simulink model "c00006M_harness"  (R2018a)
settings: Solver=FixedStepAuto  StartTime=0.0  StopTime=300  FixedStep=0.1  RelTol=1e-3
undefined symbols (not defined in the file): A1, hmax, PriorityTank, R1, R2, sigbuilder_block, TempThreshold
(part 6 of 66)

== system c00006M_harness/M105 ==
  note: VALUES
      | ---------------------------------
      | ControlType = 1 | 2 | 3
      | FillTank = 0 | 1
      | EmptyTank = 0 | 1
      | ManualReference between 0 and 1
      | Tempreature between 0 and 100
      | EmergencyButton = 0 | 1
      | LiquidLevel between 0 and 1 (hmax)
  note: Inputs For Tank2
  note: NAMES
      | --------------------------------------------
      | CT1 = ControlType Tank 1
      | F1 = Fill Tank 1
      | E1 = Empty Tank 1
      | MR1 = Manual Reference Tank1
      | T1 = Temperature Tank 1
      | EB1 = Emergency Button Tank 1
      | LL1 = Liquid Level 1
  note: Inputs For Tank3
  note: Inputs For Tank1
  CT2 : Inport
  F2 : Inport  Port=2
  E2 : Inport  Port=3
  MR2 : Inport  Port=4
  T2 : Inport  Port=5
  EB2 : Inport  Port=6
  CT3 : Inport  Port=7
  F3 : Inport  Port=8
  E3 : Inport  Port=9
  MR3 : Inport  Port=10
  T3 : Inport  Port=11
  EB3 : Inport  Port=12
  Tank2 : Subsystem
  Tank3 : Subsystem
  LL2 : Outport
  LL3 : Outport  Port=2
  wires:
  Tank2/1(LL2) -> LL2/1, Tank3/7(LL2)
  Tank3/1(LL3) -> LL3/1, Tank2/7(LL3)
  EB2/1 -> Tank2/6(EB2)
  MR3/1 -> Tank3/4(MR3)
  CT2/1 -> Tank2/1(CT2)
  F2/1 -> Tank2/2(F2)
  E3/1 -> Tank3/3(E3)
  E2/1 -> Tank2/3(E2)
  T2/1 -> Tank2/5(T2)
  CT3/1 -> Tank3/1(CT3)
  F3/1 -> Tank3/2(F3)
  EB3/1 -> Tank3/6(EB3)
  T3/1 -> Tank3/5(T3)
  MR2/1 -> Tank2/4(MR2)

== system c00006M_harness/M106 ==
  note: VALUES
      | ---------------------------------
      | ControlType = 1 | 2 | 3
      | FillTank = 0 | 1
      | EmptyTank = 0 | 1
      | ManualReference between 0 and 1
      | Tempreature between 0 and 100
      | EmergencyButton = 0 | 1
      | LiquidLevel between 0 and 1 (hmax)
  note: Inputs For Tank2
  note: NAMES
      | --------------------------------------------
      | CT1 = ControlType Tank 1
      | F1 = Fill Tank 1
      | E1 = Empty Tank 1
      | MR1 = Manual Reference Tank1
      | T1 = Temperature Tank 1
      | EB1 = Emergency Button Tank 1
      | LL1 = Liquid Level 1
  note: Inputs For Tank3
  note: Inputs For Tank1
  CT2 : Inport
  F2 : Inport  Port=2
  E2 : Inport  Port=3
  MR2 : Inport  Port=4
  T2 : Inport  Port=5
  EB2 : Inport  Port=6
  CT3 : Inport  Port=7
  F3 : Inport  Port=8
  E3 : Inport  Port=9
  MR3 : Inport  Port=10
  T3 : Inport  Port=11
  EB3 : Inport  Port=12
  Tank2 : Subsystem
  Tank3 : Subsystem
  LL2 : Outport
  LL3 : Outport  Port=2
  wires:
  Tank2/1(LL2) -> LL2/1, Tank3/7(LL2)
  Tank3/1(LL3) -> LL3/1, Tank2/7(LL3)
  EB2/1 -> Tank2/6(EB2)
  MR3/1 -> Tank3/4(MR3)
  CT2/1 -> Tank2/1(CT2)
  F2/1 -> Tank2/2(F2)
  E3/1 -> Tank3/3(E3)
  E2/1 -> Tank2/3(E2)
  T2/1 -> Tank2/5(T2)
  CT3/1 -> Tank3/1(CT3)
  F3/1 -> Tank3/2(F3)
  EB3/1 -> Tank3/6(EB3)
  T3/1 -> Tank3/5(T3)
  MR2/1 -> Tank2/4(MR2)

== system c00006M_harness/M107 ==
  note: VALUES
      | ---------------------------------
      | ControlType = 1 | 2 | 3
      | FillTank = 0 | 1
      | EmptyTank = 0 | 1
      | ManualReference between 0 and 1
      | Tempreature between 0 and 100
      | EmergencyButton = 0 | 1
      | LiquidLevel between 0 and 1 (hmax)
  note: Inputs For Tank2
  note: NAMES
      | --------------------------------------------
      | CT1 = ControlType Tank 1
      | F1 = Fill Tank 1
      | E1 = Empty Tank 1
      | MR1 = Manual Reference Tank1
      | T1 = Temperature Tank 1
      | EB1 = Emergency Button Tank 1
      | LL1 = Liquid Level 1
  note: Inputs For Tank3
  note: Inputs For Tank1
  CT2 : Inport
  F2 : Inport  Port=2
  E2 : Inport  Port=3
  MR2 : Inport  Port=4
  T2 : Inport  Port=5
  EB2 : Inport  Port=6
  CT3 : Inport  Port=7
  F3 : Inport  Port=8
  E3 : Inport  Port=9
  MR3 : Inport  Port=10
  T3 : Inport  Port=11
  EB3 : Inport  Port=12
  Tank2 : Subsystem
  Tank3 : Subsystem
  LL2 : Outport
  LL3 : Outport  Port=2
  wires:
  Tank2/1(LL2) -> LL2/1, Tank3/7(LL2)
  Tank3/1(LL3) -> LL3/1, Tank2/7(LL3)
  EB2/1 -> Tank2/6(EB2)
  MR3/1 -> Tank3/4(MR3)
  CT2/1 -> Tank2/1(CT2)
  F2/1 -> Tank2/2(F2)
  E3/1 -> Tank3/3(E3)
  E2/1 -> Tank2/3(E2)
  T2/1 -> Tank2/5(T2)
  CT3/1 -> Tank3/1(CT3)
  F3/1 -> Tank3/2(F3)
  EB3/1 -> Tank3/6(EB3)
  T3/1 -> Tank3/5(T3)
  MR2/1 -> Tank2/4(MR2)

== system c00006M_harness/M108 ==
  note: VALUES
      | ---------------------------------
      | ControlType = 1 | 2 | 3
      | FillTank = 0 | 1
      | EmptyTank = 0 | 1
      | ManualReference between 0 and 1
      | Tempreature between 0 and 100
      | EmergencyButton = 0 | 1
      | LiquidLevel between 0 and 1 (hmax)
  note: Inputs For Tank2
  note: NAMES
      | --------------------------------------------
      | CT1 = ControlType Tank 1
      | F1 = Fill Tank 1
      | E1 = Empty Tank 1
      | MR1 = Manual Reference Tank1
      | T1 = Temperature Tank 1
      | EB1 = Emergency Button Tank 1
      | LL1 = Liquid Level 1
  note: Inputs For Tank3
  note: Inputs For Tank1
  CT2 : Inport
  F2 : Inport  Port=2
  E2 : Inport  Port=3
  MR2 : Inport  Port=4
  T2 : Inport  Port=5
  EB2 : Inport  Port=6
  CT3 : Inport  Port=7
  F3 : Inport  Port=8
  E3 : Inport  Port=9
  MR3 : Inport  Port=10
  T3 : Inport  Port=11
  EB3 : Inport  Port=12
  Tank2 : Subsystem
  Tank3 : Subsystem
  LL2 : Outport
  LL3 : Outport  Port=2
  wires:
  Tank2/1(LL2) -> LL2/1, Tank3/7(LL2)
  Tank3/1(LL3) -> LL3/1, Tank2/7(LL3)
  EB2/1 -> Tank2/6(EB2)
  MR3/1 -> Tank3/4(MR3)
  CT2/1 -> Tank2/1(CT2)
  F2/1 -> Tank2/2(F2)
  E3/1 -> Tank3/3(E3)
  E2/1 -> Tank2/3(E2)
  T2/1 -> Tank2/5(T2)
  CT3/1 -> Tank3/1(CT3)
  F3/1 -> Tank3/2(F3)
  EB3/1 -> Tank3/6(EB3)
  T3/1 -> Tank3/5(T3)
  MR2/1 -> Tank2/4(MR2)

== system c00006M_harness/M109 ==
  note: VALUES
      | ---------------------------------
      | ControlType = 1 | 2 | 3
      | FillTank = 0 | 1
      | EmptyTank = 0 | 1
      | ManualReference between 0 and 1
      | Tempreature between 0 and 100
      | EmergencyButton = 0 | 1
      | LiquidLevel between 0 and 1 (hmax)
  note: Inputs For Tank2
  note: NAMES
      | --------------------------------------------
      | CT1 = ControlType Tank 1
      | F1 = Fill Tank 1
      | E1 = Empty Tank 1
      | MR1 = Manual Reference Tank1
      | T1 = Temperature Tank 1
      | EB1 = Emergency Button Tank 1
      | LL1 = Liquid Level 1
  note: Inputs For Tank3
  note: Inputs For Tank1
  CT2 : Inport
  F2 : Inport  Port=2
  E2 : Inport  Port=3
  MR2 : Inport  Port=4
  T2 : Inport  Port=5
  EB2 : Inport  Port=6
  CT3 : Inport  Port=7
  F3 : Inport  Port=8
  E3 : Inport  Port=9
  MR3 : Inport  Port=10
  T3 : Inport  Port=11
  EB3 : Inport  Port=12
  Tank2 : Subsystem
  Tank3 : Subsystem
  LL2 : Outport
  LL3 : Outport  Port=2
  wires:
  Tank2/1(LL2) -> LL2/1, Tank3/7(LL2)
  Tank3/1(LL3) -> LL3/1, Tank2/7(LL3)
  EB2/1 -> Tank2/6(EB2)
  MR3/1 -> Tank3/4(MR3)
  CT2/1 -> Tank2/1(CT2)
  F2/1 -> Tank2/2(F2)
  E3/1 -> Tank3/3(E3)
  E2/1 -> Tank2/3(E2)
  T2/1 -> Tank2/5(T2)
  CT3/1 -> Tank3/1(CT3)
  F3/1 -> Tank3/2(F3)
  EB3/1 -> Tank3/6(EB3)
  T3/1 -> Tank3/5(T3)
  MR2/1 -> Tank2/4(MR2)

== system c00006M_harness/M110 ==
  note: VALUES
      | ---------------------------------
      | ControlType = 1 | 2 | 3
      | FillTank = 0 | 1
      | EmptyTank = 0 | 1
      | ManualReference between 0 and 1
      | Tempreature between 0 and 100
      | EmergencyButton = 0 | 1
      | LiquidLevel between 0 and 1 (hmax)
  note: Inputs For Tank2
  note: NAMES
      | --------------------------------------------
      | CT1 = ControlType Tank 1
      | F1 = Fill Tank 1
      | E1 = Empty Tank 1
      | MR1 = Manual Reference Tank1
      | T1 = Temperature Tank 1
      | EB1 = Emergency Button Tank 1
      | LL1 = Liquid Level 1
  note: Inputs For Tank3
  note: Inputs For Tank1
  CT2 : Inport
  F2 : Inport  Port=2
  E2 : Inport  Port=3
  MR2 : Inport  Port=4
  T2 : Inport  Port=5
  EB2 : Inport  Port=6
  CT3 : Inport  Port=7
  F3 : Inport  Port=8
  E3 : Inport  Port=9
  MR3 : Inport  Port=10
  T3 : Inport  Port=11
  EB3 : Inport  Port=12
  Tank2 : Subsystem
  Tank3 : Subsystem
  LL2 : Outport
  LL3 : Outport  Port=2
  wires:
  Tank2/1(LL2) -> LL2/1, Tank3/7(LL2)
  Tank3/1(LL3) -> LL3/1, Tank2/7(LL3)
  EB2/1 -> Tank2/6(EB2)
  MR3/1 -> Tank3/4(MR3)
  CT2/1 -> Tank2/1(CT2)
  F2/1 -> Tank2/2(F2)
  E3/1 -> Tank3/3(E3)
  E2/1 -> Tank2/3(E2)
  T2/1 -> Tank2/5(T2)
  CT3/1 -> Tank3/1(CT3)
  F3/1 -> Tank3/2(F3)
  EB3/1 -> Tank3/6(EB3)
  T3/1 -> Tank3/5(T3)
  MR2/1 -> Tank2/4(MR2)

== system c00006M_harness/M111 ==
  note: VALUES
      | ---------------------------------
      | ControlType = 1 | 2 | 3
      | FillTank = 0 | 1
      | EmptyTank = 0 | 1
      | ManualReference between 0 and 1
      | Tempreature between 0 and 100
      | EmergencyButton = 0 | 1
      | LiquidLevel between 0 and 1 (hmax)
  note: Inputs For Tank2
  note: NAMES
      | --------------------------------------------
      | CT1 = ControlType Tank 1
      | F1 = Fill Tank 1
      | E1 = Empty Tank 1
      | MR1 = Manual Reference Tank1
      | T1 = Temperature Tank 1
      | EB1 = Emergency Button Tank 1
      | LL1 = Liquid Level 1
  note: Inputs For Tank3
  note: Inputs For Tank1
  CT2 : Inport
  F2 : Inport  Port=2
  E2 : Inport  Port=3
  MR2 : Inport  Port=4
  T2 : Inport  Port=5
  EB2 : Inport  Port=6
  CT3 : Inport  Port=7
  F3 : Inport  Port=8
  E3 : Inport  Port=9
  MR3 : Inport  Port=10
  T3 : Inport  Port=11
  EB3 : Inport  Port=12
  Tank2 : Subsystem
  Tank3 : Subsystem
  LL2 : Outport
  LL3 : Outport  Port=2
  wires:
  Tank2/1(LL2) -> LL2/1, Tank3/7(LL2)
  Tank3/1(LL3) -> LL3/1, Tank2/7(LL3)
  EB2/1 -> Tank2/6(EB2)
  MR3/1 -> Tank3/4(MR3)
  CT2/1 -> Tank2/1(CT2)
  F2/1 -> Tank2/2(F2)
  E3/1 -> Tank3/3(E3)
  E2/1 -> Tank2/3(E2)
  T2/1 -> Tank2/5(T2)
  CT3/1 -> Tank3/1(CT3)
  F3/1 -> Tank3/2(F3)
  EB3/1 -> Tank3/6(EB3)
  T3/1 -> Tank3/5(T3)
  MR2/1 -> Tank2/4(MR2)

== system c00006M_harness/M112 ==
  note: VALUES
      | ---------------------------------
      | ControlType = 1 | 2 | 3
      | FillTank = 0 | 1
      | EmptyTank = 0 | 1
      | ManualReference between 0 and 1
      | Tempreature between 0 and 100
      | EmergencyButton = 0 | 1
      | LiquidLevel between 0 and 1 (hmax)
  note: Inputs For Tank2
  note: NAMES
      | --------------------------------------------
      | CT1 = ControlType Tank 1
      | F1 = Fill Tank 1
      | E1 = Empty Tank 1
      | MR1 = Manual Reference Tank1
      | T1 = Temperature Tank 1
      | EB1 = Emergency Button Tank 1
      | LL1 = Liquid Level 1
  note: Inputs For Tank3
  note: Inputs For Tank1
  CT2 : Inport
  F2 : Inport  Port=2
  E2 : Inport  Port=3
  MR2 : Inport  Port=4
  T2 : Inport  Port=5
  EB2 : Inport  Port=6
  CT3 : Inport  Port=7
  F3 : Inport  Port=8
  E3 : Inport  Port=9
  MR3 : Inport  Port=10
  T3 : Inport  Port=11
  EB3 : Inport  Port=12
  Tank2 : Subsystem
  Tank3 : Subsystem
  LL2 : Outport
  LL3 : Outport  Port=2
  wires:
  Tank2/1(LL2) -> LL2/1, Tank3/7(LL2)
  Tank3/1(LL3) -> LL3/1, Tank2/7(LL3)
  EB2/1 -> Tank2/6(EB2)
  MR3/1 -> Tank3/4(MR3)
  CT2/1 -> Tank2/1(CT2)
  F2/1 -> Tank2/2(F2)
  E3/1 -> Tank3/3(E3)
  E2/1 -> Tank2/3(E2)
  T2/1 -> Tank2/5(T2)
  CT3/1 -> Tank3/1(CT3)
  F3/1 -> Tank3/2(F3)
  EB3/1 -> Tank3/6(EB3)
  T3/1 -> Tank3/5(T3)
  MR2/1 -> Tank2/4(MR2)

== system c00006M_harness/M113 ==
  note: VALUES
      | ---------------------------------
      | ControlType = 1 | 2 | 3
      | FillTank = 0 | 1
      | EmptyTank = 0 | 1
      | ManualReference between 0 and 1
      | Tempreature between 0 and 100
      | EmergencyButton = 0 | 1
      | LiquidLevel between 0 and 1 (hmax)
  note: Inputs For Tank2
  note: NAMES
      | --------------------------------------------
      | CT1 = ControlType Tank 1
      | F1 = Fill Tank 1
      | E1 = Empty Tank 1
      | MR1 = Manual Reference Tank1
      | T1 = Temperature Tank 1
      | EB1 = Emergency Button Tank 1
      | LL1 = Liquid Level 1
  note: Inputs For Tank3
  note: Inputs For Tank1
  CT2 : Inport
  F2 : Inport  Port=2
  E2 : Inport  Port=3
  MR2 : Inport  Port=4
  T2 : Inport  Port=5
  EB2 : Inport  Port=6
  CT3 : Inport  Port=7
  F3 : Inport  Port=8
  E3 : Inport  Port=9
  MR3 : Inport  Port=10
  T3 : Inport  Port=11
  EB3 : Inport  Port=12
  Tank2 : Subsystem
  Tank3 : Subsystem
  LL2 : Outport
  LL3 : Outport  Port=2
  wires:
  Tank2/1(LL2) -> LL2/1, Tank3/7(LL2)
  Tank3/1(LL3) -> LL3/1, Tank2/7(LL3)
  EB2/1 -> Tank2/6(EB2)
  MR3/1 -> Tank3/4(MR3)
  CT2/1 -> Tank2/1(CT2)
  F2/1 -> Tank2/2(F2)
  E3/1 -> Tank3/3(E3)
  E2/1 -> Tank2/3(E2)
  T2/1 -> Tank2/5(T2)
  CT3/1 -> Tank3/1(CT3)
  F3/1 -> Tank3/2(F3)
  EB3/1 -> Tank3/6(EB3)
  T3/1 -> Tank3/5(T3)
  MR2/1 -> Tank2/4(MR2)

== system c00006M_harness/M114 ==
  note: VALUES
      | ---------------------------------
      | ControlType = 1 | 2 | 3
      | FillTank = 0 | 1
      | EmptyTank = 0 | 1
      | ManualReference between 0 and 1
      | Tempreature between 0 and 100
      | EmergencyButton = 0 | 1
      | LiquidLevel between 0 and 1 (hmax)
  note: Inputs For Tank2
  note: NAMES
      | --------------------------------------------
      | CT1 = ControlType Tank 1
      | F1 = Fill Tank 1
      | E1 = Empty Tank 1
      | MR1 = Manual Reference Tank1
      | T1 = Temperature Tank 1
      | EB1 = Emergency Button Tank 1
      | LL1 = Liquid Level 1
  note: Inputs For Tank3
  note: Inputs For Tank1
  CT2 : Inport
  F2 : Inport  Port=2
  E2 : Inport  Port=3
  MR2 : Inport  Port=4
  T2 : Inport  Port=5
  EB2 : Inport  Port=6
  CT3 : Inport  Port=7
  F3 : Inport  Port=8
  E3 : Inport  Port=9
  MR3 : Inport  Port=10
  T3 : Inport  Port=11
  EB3 : Inport  Port=12
  Tank2 : Subsystem
  Tank3 : Subsystem
  LL2 : Outport
  LL3 : Outport  Port=2
  wires:
  Tank2/1(LL2) -> LL2/1, Tank3/7(LL2)
  Tank3/1(LL3) -> LL3/1, Tank2/7(LL3)
  EB2/1 -> Tank2/6(EB2)
  MR3/1 -> Tank3/4(MR3)
  CT2/1 -> Tank2/1(CT2)
  F2/1 -> Tank2/2(F2)
  E3/1 -> Tank3/3(E3)
  E2/1 -> Tank2/3(E2)
  T2/1 -> Tank2/5(T2)
  CT3/1 -> Tank3/1(CT3)
  F3/1 -> Tank3/2(F3)
  EB3/1 -> Tank3/6(EB3)
  T3/1 -> Tank3/5(T3)
  MR2/1 -> Tank2/4(MR2)

== system c00006M_harness/M115 ==
  note: VALUES
      | ---------------------------------
      | ControlType = 1 | 2 | 3
      | FillTank = 0 | 1
      | EmptyTank = 0 | 1
      | ManualReference between 0 and 1
      | Tempreature between 0 and 100
      | EmergencyButton = 0 | 1
      | LiquidLevel between 0 and 1 (hmax)
  note: Inputs For Tank2
  note: NAMES
      | --------------------------------------------
      | CT1 = ControlType Tank 1
      | F1 = Fill Tank 1
      | E1 = Empty Tank 1
      | MR1 = Manual Reference Tank1
      | T1 = Temperature Tank 1
      | EB1 = Emergency Button Tank 1
      | LL1 = Liquid Level 1
  note: Inputs For Tank3
  note: Inputs For Tank1
  CT2 : Inport
  F2 : Inport  Port=2
  E2 : Inport  Port=3
  MR2 : Inport  Port=4
  T2 : Inport  Port=5
  EB2 : Inport  Port=6
  CT3 : Inport  Port=7
  F3 : Inport  Port=8
  E3 : Inport  Port=9
  MR3 : Inport  Port=10
  T3 : Inport  Port=11
  EB3 : Inport  Port=12
  Tank2 : Subsystem
  Tank3 : Subsystem
  LL2 : Outport
  LL3 : Outport  Port=2
  wires:
  Tank2/1(LL2) -> LL2/1, Tank3/7(LL2)
  Tank3/1(LL3) -> LL3/1, Tank2/7(LL3)
  EB2/1 -> Tank2/6(EB2)
  MR3/1 -> Tank3/4(MR3)
  CT2/1 -> Tank2/1(CT2)
  F2/1 -> Tank2/2(F2)
  E3/1 -> Tank3/3(E3)
  E2/1 -> Tank2/3(E2)
  T2/1 -> Tank2/5(T2)
  CT3/1 -> Tank3/1(CT3)
  F3/1 -> Tank3/2(F3)
  EB3/1 -> Tank3/6(EB3)
  T3/1 -> Tank3/5(T3)
  MR2/1 -> Tank2/4(MR2)

== system c00006M_harness/M116 ==
  note: VALUES
      | ---------------------------------
      | ControlType = 1 | 2 | 3
      | FillTank = 0 | 1
      | EmptyTank = 0 | 1
      | ManualReference between 0 and 1
      | Tempreature between 0 and 100
      | EmergencyButton = 0 | 1
      | LiquidLevel between 0 and 1 (hmax)
  note: Inputs For Tank2
  note: NAMES
      | --------------------------------------------
      | CT1 = ControlType Tank 1
      | F1 = Fill Tank 1
      | E1 = Empty Tank 1
      | MR1 = Manual Reference Tank1
      | T1 = Temperature Tank 1
      | EB1 = Emergency Button Tank 1
      | LL1 = Liquid Level 1
  note: Inputs For Tank3
  note: Inputs For Tank1
  CT2 : Inport
  F2 : Inport  Port=2
  E2 : Inport  Port=3
  MR2 : Inport  Port=4
  T2 : Inport  Port=5
  EB2 : Inport  Port=6
  CT3 : Inport  Port=7
  F3 : Inport  Port=8
  E3 : Inport  Port=9
  MR3 : Inport  Port=10
  T3 : Inport  Port=11
  EB3 : Inport  Port=12
  Tank2 : Subsystem
  Tank3 : Subsystem
  LL2 : Outport
  LL3 : Outport  Port=2
  wires:
  Tank2/1(LL2) -> LL2/1, Tank3/7(LL2)
  Tank3/1(LL3) -> LL3/1, Tank2/7(LL3)
  EB2/1 -> Tank2/6(EB2)
  MR3/1 -> Tank3/4(MR3)
  CT2/1 -> Tank2/1(CT2)
  F2/1 -> Tank2/2(F2)
  E3/1 -> Tank3/3(E3)
  E2/1 -> Tank2/3(E2)
  T2/1 -> Tank2/5(T2)
  CT3/1 -> Tank3/1(CT3)
  F3/1 -> Tank3/2(F3)
  EB3/1 -> Tank3/6(EB3)
  T3/1 -> Tank3/5(T3)
  MR2/1 -> Tank2/4(MR2)

== system c00006M_harness/M117 ==
  note: VALUES
      | ---------------------------------
      | ControlType = 1 | 2 | 3
      | FillTank = 0 | 1
      | EmptyTank = 0 | 1
      | ManualReference between 0 and 1
      | Tempreature between 0 and 100
      | EmergencyButton = 0 | 1
      | LiquidLevel between 0 and 1 (hmax)
  note: Inputs For Tank2
  note: NAMES
      | --------------------------------------------
      | CT1 = ControlType Tank 1
      | F1 = Fill Tank 1
      | E1 = Empty Tank 1
      | MR1 = Manual Reference Tank1
      | T1 = Temperature Tank 1
      | EB1 = Emergency Button Tank 1
      | LL1 = Liquid Level 1
  note: Inputs For Tank3
  note: Inputs For Tank1
  CT2 : Inport
  F2 : Inport  Port=2
  E2 : Inport  Port=3
  MR2 : Inport  Port=4
  T2 : Inport  Port=5
  EB2 : Inport  Port=6
  CT3 : Inport  Port=7
  F3 : Inport  Port=8
  E3 : Inport  Port=9
  MR3 : Inport  Port=10
  T3 : Inport  Port=11
  EB3 : Inport  Port=12
  Tank2 : Subsystem
  Tank3 : Subsystem
  LL2 : Outport
  LL3 : Outport  Port=2
  wires:
  Tank2/1(LL2) -> LL2/1, Tank3/7(LL2)
  Tank3/1(LL3) -> LL3/1, Tank2/7(LL3)
  EB2/1 -> Tank2/6(EB2)
  MR3/1 -> Tank3/4(MR3)
  CT2/1 -> Tank2/1(CT2)
  F2/1 -> Tank2/2(F2)
  E3/1 -> Tank3/3(E3)
  E2/1 -> Tank2/3(E2)
  T2/1 -> Tank2/5(T2)
  CT3/1 -> Tank3/1(CT3)
  F3/1 -> Tank3/2(F3)
  EB3/1 -> Tank3/6(EB3)
  T3/1 -> Tank3/5(T3)
  MR2/1 -> Tank2/4(MR2)

== system c00006M_harness/M118 ==
  note: VALUES
      | ---------------------------------
      | ControlType = 1 | 2 | 3
      | FillTank = 0 | 1
      | EmptyTank = 0 | 1
      | ManualReference between 0 and 1
      | Tempreature between 0 and 100
      | EmergencyButton = 0 | 1
      | LiquidLevel between 0 and 1 (hmax)
  note: Inputs For Tank2
  note: NAMES
      | --------------------------------------------
      | CT1 = ControlType Tank 1
      | F1 = Fill Tank 1
      | E1 = Empty Tank 1
      | MR1 = Manual Reference Tank1
      | T1 = Temperature Tank 1
      | EB1 = Emergency Button Tank 1
      | LL1 = Liquid Level 1
  note: Inputs For Tank3
  note: Inputs For Tank1
  CT2 : Inport
  F2 : Inport  Port=2
  E2 : Inport  Port=3
  MR2 : Inport  Port=4
  T2 : Inport  Port=5
  EB2 : Inport  Port=6
  CT3 : Inport  Port=7
  F3 : Inport  Port=8
  E3 : Inport  Port=9
  MR3 : Inport  Port=10
  T3 : Inport  Port=11
  EB3 : Inport  Port=12
  Tank2 : Subsystem
  Tank3 : Subsystem
  LL2 : Outport
  LL3 : Outport  Port=2
  wires:
  Tank2/1(LL2) -> LL2/1, Tank3/7(LL2)
  Tank3/1(LL3) -> LL3/1, Tank2/7(LL3)
  EB2/1 -> Tank2/6(EB2)
  MR3/1 -> Tank3/4(MR3)
  CT2/1 -> Tank2/1(CT2)
  F2/1 -> Tank2/2(F2)
  E3/1 -> Tank3/3(E3)
  E2/1 -> Tank2/3(E2)
  T2/1 -> Tank2/5(T2)
  CT3/1 -> Tank3/1(CT3)
  F3/1 -> Tank3/2(F3)
  EB3/1 -> Tank3/6(EB3)
  T3/1 -> Tank3/5(T3)
  MR2/1 -> Tank2/4(MR2)

== system c00006M_harness/M119 ==
  note: VALUES
      | ---------------------------------
      | ControlType = 1 | 2 | 3
      | FillTank = 0 | 1
      | EmptyTank = 0 | 1
      | ManualReference between 0 and 1
      | Tempreature between 0 and 100
      | EmergencyButton = 0 | 1
      | LiquidLevel between 0 and 1 (hmax)
  note: Inputs For Tank2
  note: NAMES
      | --------------------------------------------
      | CT1 = ControlType Tank 1
      | F1 = Fill Tank 1
      | E1 = Empty Tank 1
      | MR1 = Manual Reference Tank1
      | T1 = Temperature Tank 1
      | EB1 = Emergency Button Tank 1
      | LL1 = Liquid Level 1
  note: Inputs For Tank3
  note: Inputs For Tank1
  CT2 : Inport
  F2 : Inport  Port=2
  E2 : Inport  Port=3
  MR2 : Inport  Port=4
  T2 : Inport  Port=5
  EB2 : Inport  Port=6
  CT3 : Inport  Port=7
  F3 : Inport  Port=8
  E3 : Inport  Port=9
  MR3 : Inport  Port=10
  T3 : Inport  Port=11
  EB3 : Inport  Port=12
  Tank2 : Subsystem
  Tank3 : Subsystem
  LL2 : Outport
  LL3 : Outport  Port=2
  wires:
  Tank2/1(LL2) -> LL2/1, Tank3/7(LL2)
  Tank3/1(LL3) -> LL3/1, Tank2/7(LL3)
  EB2/1 -> Tank2/6(EB2)
  MR3/1 -> Tank3/4(MR3)
  CT2/1 -> Tank2/1(CT2)
  F2/1 -> Tank2/2(F2)
  E3/1 -> Tank3/3(E3)
  E2/1 -> Tank2/3(E2)
  T2/1 -> Tank2/5(T2)
  CT3/1 -> Tank3/1(CT3)
  F3/1 -> Tank3/2(F3)
  EB3/1 -> Tank3/6(EB3)
  T3/1 -> Tank3/5(T3)
  MR2/1 -> Tank2/4(MR2)

== system c00006M_harness/M120 ==
  note: VALUES
      | ---------------------------------
      | ControlType = 1 | 2 | 3
      | FillTank = 0 | 1
      | EmptyTank = 0 | 1
      | ManualReference between 0 and 1
      | Tempreature between 0 and 100
      | EmergencyButton = 0 | 1
      | LiquidLevel between 0 and 1 (hmax)
  note: Inputs For Tank2
  note: NAMES
      | --------------------------------------------
      | CT1 = ControlType Tank 1
      | F1 = Fill Tank 1
      | E1 = Empty Tank 1
      | MR1 = Manual Reference Tank1
      | T1 = Temperature Tank 1
      | EB1 = Emergency Button Tank 1
      | LL1 = Liquid Level 1
  note: Inputs For Tank3
  note: Inputs For Tank1
  CT2 : Inport
  F2 : Inport  Port=2
  E2 : Inport  Port=3
  MR2 : Inport  Port=4
  T2 : Inport  Port=5
  EB2 : Inport  Port=6
  CT3 : Inport  Port=7
  F3 : Inport  Port=8
  E3 : Inport  Port=9
  MR3 : Inport  Port=10
  T3 : Inport  Port=11
  EB3 : Inport  Port=12
  Tank2 : Subsystem
  Tank3 : Subsystem
  LL2 : Outport
  LL3 : Outport  Port=2
  wires:
  Tank2/1(LL2) -> LL2/1, Tank3/7(LL2)
  Tank3/1(LL3) -> LL3/1, Tank2/7(LL3)
  EB2/1 -> Tank2/6(EB2)
  MR3/1 -> Tank3/4(MR3)
  CT2/1 -> Tank2/1(CT2)
  F2/1 -> Tank2/2(F2)
  E3/1 -> Tank3/3(E3)
  E2/1 -> Tank2/3(E2)
  T2/1 -> Tank2/5(T2)
  CT3/1 -> Tank3/1(CT3)
  F3/1 -> Tank3/2(F3)
  EB3/1 -> Tank3/6(EB3)
  T3/1 -> Tank3/5(T3)
  MR2/1 -> Tank2/4(MR2)

== system c00006M_harness/M121 ==
  note: VALUES
      | ---------------------------------
      | ControlType = 1 | 2 | 3
      | FillTank = 0 | 1
      | EmptyTank = 0 | 1
      | ManualReference between 0 and 1
      | Tempreature between 0 and 100
      | EmergencyButton = 0 | 1
      | LiquidLevel between 0 and 1 (hmax)
  note: Inputs For Tank2
  note: NAMES
      | --------------------------------------------
      | CT1 = ControlType Tank 1
      | F1 = Fill Tank 1
      | E1 = Empty Tank 1
      | MR1 = Manual Reference Tank1
      | T1 = Temperature Tank 1
      | EB1 = Emergency Button Tank 1
      | LL1 = Liquid Level 1
  note: Inputs For Tank3
  note: Inputs For Tank1
  CT2 : Inport
  F2 : Inport  Port=2
  E2 : Inport  Port=3
  MR2 : Inport  Port=4
  T2 : Inport  Port=5
  EB2 : Inport  Port=6
  CT3 : Inport  Port=7
  F3 : Inport  Port=8
  E3 : Inport  Port=9
  MR3 : Inport  Port=10
  T3 : Inport  Port=11
  EB3 : Inport  Port=12
  Tank2 : Subsystem
  Tank3 : Subsystem
  LL2 : Outport
  LL3 : Outport  Port=2
  wires:
  Tank2/1(LL2) -> LL2/1, Tank3/7(LL2)
  Tank3/1(LL3) -> LL3/1, Tank2/7(LL3)
  EB2/1 -> Tank2/6(EB2)
  MR3/1 -> Tank3/4(MR3)
  CT2/1 -> Tank2/1(CT2)
  F2/1 -> Tank2/2(F2)
  E3/1 -> Tank3/3(E3)
  E2/1 -> Tank2/3(E2)
  T2/1 -> Tank2/5(T2)
  CT3/1 -> Tank3/1(CT3)
  F3/1 -> Tank3/2(F3)
  EB3/1 -> Tank3/6(EB3)
  T3/1 -> Tank3/5(T3)
  MR2/1 -> Tank2/4(MR2)

== system c00006M_harness/M122 ==
  note: VALUES
      | ---------------------------------
      | ControlType = 1 | 2 | 3
      | FillTank = 0 | 1
      | EmptyTank = 0 | 1
      | ManualReference between 0 and 1
      | Tempreature between 0 and 100
      | EmergencyButton = 0 | 1
      | LiquidLevel between 0 and 1 (hmax)
  note: Inputs For Tank2
  note: NAMES
      | --------------------------------------------
      | CT1 = ControlType Tank 1
      | F1 = Fill Tank 1
      | E1 = Empty Tank 1
      | MR1 = Manual Reference Tank1
      | T1 = Temperature Tank 1
      | EB1 = Emergency Button Tank 1
      | LL1 = Liquid Level 1
  note: Inputs For Tank3
  note: Inputs For Tank1
  CT2 : Inport
  F2 : Inport  Port=2
  E2 : Inport  Port=3
  MR2 : Inport  Port=4
  T2 : Inport  Port=5
  EB2 : Inport  Port=6
  CT3 : Inport  Port=7
  F3 : Inport  Port=8
  E3 : Inport  Port=9
  MR3 : Inport  Port=10
  T3 : Inport  Port=11
  EB3 : Inport  Port=12
  Tank2 : Subsystem
  Tank3 : Subsystem
  LL2 : Outport
  LL3 : Outport  Port=2
  wires:
  Tank2/1(LL2) -> LL2/1, Tank3/7(LL2)
  Tank3/1(LL3) -> LL3/1, Tank2/7(LL3)
  EB2/1 -> Tank2/6(EB2)
  MR3/1 -> Tank3/4(MR3)
  CT2/1 -> Tank2/1(CT2)
  F2/1 -> Tank2/2(F2)
  E3/1 -> Tank3/3(E3)
  E2/1 -> Tank2/3(E2)
  T2/1 -> Tank2/5(T2)
  CT3/1 -> Tank3/1(CT3)
  F3/1 -> Tank3/2(F3)
  EB3/1 -> Tank3/6(EB3)
  T3/1 -> Tank3/5(T3)
  MR2/1 -> Tank2/4(MR2)

== system c00006M_harness/M123 ==
  note: VALUES
      | ---------------------------------
      | ControlType = 1 | 2 | 3
      | FillTank = 0 | 1
      | EmptyTank = 0 | 1
      | ManualReference between 0 and 1
      | Tempreature between 0 and 100
      | EmergencyButton = 0 | 1
      | LiquidLevel between 0 and 1 (hmax)
  note: Inputs For Tank2
  note: NAMES
      | --------------------------------------------
      | CT1 = ControlType Tank 1
      | F1 = Fill Tank 1
      | E1 = Empty Tank 1
      | MR1 = Manual Reference Tank1
      | T1 = Temperature Tank 1
      | EB1 = Emergency Button Tank 1
      | LL1 = Liquid Level 1
  note: Inputs For Tank3
  note: Inputs For Tank1
  CT2 : Inport
  F2 : Inport  Port=2
  E2 : Inport  Port=3
  MR2 : Inport  Port=4
  T2 : Inport  Port=5
  EB2 : Inport  Port=6
  CT3 : Inport  Port=7
  F3 : Inport  Port=8
  E3 : Inport  Port=9
  MR3 : Inport  Port=10
  T3 : Inport  Port=11
  EB3 : Inport  Port=12
  Tank2 : Subsystem
  Tank3 : Subsystem
  LL2 : Outport
  LL3 : Outport  Port=2
  wires:
  Tank2/1(LL2) -> LL2/1, Tank3/7(LL2)
  Tank3/1(LL3) -> LL3/1, Tank2/7(LL3)
  EB2/1 -> Tank2/6(EB2)
  MR3/1 -> Tank3/4(MR3)
  CT2/1 -> Tank2/1(CT2)
  F2/1 -> Tank2/2(F2)
  E3/1 -> Tank3/3(E3)
  E2/1 -> Tank2/3(E2)
  T2/1 -> Tank2/5(T2)
  CT3/1 -> Tank3/1(CT3)
  F3/1 -> Tank3/2(F3)
  EB3/1 -> Tank3/6(EB3)
  T3/1 -> Tank3/5(T3)
  MR2/1 -> Tank2/4(MR2)

== system c00006M_harness/M124 ==
  note: VALUES
      | ---------------------------------
      | ControlType = 1 | 2 | 3
      | FillTank = 0 | 1
      | EmptyTank = 0 | 1
      | ManualReference between 0 and 1
      | Tempreature between 0 and 100
      | EmergencyButton = 0 | 1
      | LiquidLevel between 0 and 1 (hmax)
  note: Inputs For Tank2
  note: NAMES
      | --------------------------------------------
      | CT1 = ControlType Tank 1
      | F1 = Fill Tank 1
      | E1 = Empty Tank 1
      | MR1 = Manual Reference Tank1
      | T1 = Temperature Tank 1
      | EB1 = Emergency Button Tank 1
      | LL1 = Liquid Level 1
  note: Inputs For Tank3
  note: Inputs For Tank1
  CT2 : Inport
  F2 : Inport  Port=2
  E2 : Inport  Port=3
  MR2 : Inport  Port=4
  T2 : Inport  Port=5
  EB2 : Inport  Port=6
  CT3 : Inport  Port=7
  F3 : Inport  Port=8
  E3 : Inport  Port=9
  MR3 : Inport  Port=10
  T3 : Inport  Port=11
  EB3 : Inport  Port=12
  Tank2 : Subsystem
  Tank3 : Subsystem
  LL2 : Outport
  LL3 : Outport  Port=2
  wires:
  Tank2/1(LL2) -> LL2/1, Tank3/7(LL2)
  Tank3/1(LL3) -> LL3/1, Tank2/7(LL3)
  EB2/1 -> Tank2/6(EB2)
  MR3/1 -> Tank3/4(MR3)
  CT2/1 -> Tank2/1(CT2)
  F2/1 -> Tank2/2(F2)
  E3/1 -> Tank3/3(E3)
  E2/1 -> Tank2/3(E2)
  T2/1 -> Tank2/5(T2)
  CT3/1 -> Tank3/1(CT3)
  F3/1 -> Tank3/2(F3)
  EB3/1 -> Tank3/6(EB3)
  T3/1 -> Tank3/5(T3)
  MR2/1 -> Tank2/4(MR2)

== system c00006M_harness/M125 ==
  note: VALUES
      | ---------------------------------
      | ControlType = 1 | 2 | 3
      | FillTank = 0 | 1
      | EmptyTank = 0 | 1
      | ManualReference between 0 and 1
      | Tempreature between 0 and 100
      | EmergencyButton = 0 | 1
      | LiquidLevel between 0 and 1 (hmax)
  note: Inputs For Tank2
  note: NAMES
      | --------------------------------------------
      | CT1 = ControlType Tank 1
      | F1 = Fill Tank 1
      | E1 = Empty Tank 1
      | MR1 = Manual Reference Tank1
      | T1 = Temperature Tank 1
      | EB1 = Emergency Button Tank 1
      | LL1 = Liquid Level 1
  note: Inputs For Tank3
  note: Inputs For Tank1
  CT2 : Inport
  F2 : Inport  Port=2
  E2 : Inport  Port=3
  MR2 : Inport  Port=4
  T2 : Inport  Port=5
  EB2 : Inport  Port=6
  CT3 : Inport  Port=7
  F3 : Inport  Port=8
  E3 : Inport  Port=9
  MR3 : Inport  Port=10
  T3 : Inport  Port=11
  EB3 : Inport  Port=12
  Tank2 : Subsystem
  Tank3 : Subsystem
  LL2 : Outport
  LL3 : Outport  Port=2
  wires:
  Tank2/1(LL2) -> LL2/1, Tank3/7(LL2)
  Tank3/1(LL3) -> LL3/1, Tank2/7(LL3)
  EB2/1 -> Tank2/6(EB2)
  MR3/1 -> Tank3/4(MR3)
  CT2/1 -> Tank2/1(CT2)
  F2/1 -> Tank2/2(F2)
  E3/1 -> Tank3/3(E3)
  E2/1 -> Tank2/3(E2)
  T2/1 -> Tank2/5(T2)
  CT3/1 -> Tank3/1(CT3)
  F3/1 -> Tank3/2(F3)
  EB3/1 -> Tank3/6(EB3)
  T3/1 -> Tank3/5(T3)
  MR2/1 -> Tank2/4(MR2)

== system c00006M_harness/M126 ==
  note: VALUES
      | ---------------------------------
      | ControlType = 1 | 2 | 3
      | FillTank = 0 | 1
      | EmptyTank = 0 | 1
      | ManualReference between 0 and 1
      | Tempreature between 0 and 100
      | EmergencyButton = 0 | 1
      | LiquidLevel between 0 and 1 (hmax)
  note: Inputs For Tank2
  note: NAMES
      | --------------------------------------------
      | CT1 = ControlType Tank 1
      | F1 = Fill Tank 1
      | E1 = Empty Tank 1
      | MR1 = Manual Reference Tank1
      | T1 = Temperature Tank 1
      | EB1 = Emergency Button Tank 1
      | LL1 = Liquid Level 1
  note: Inputs For Tank3
  note: Inputs For Tank1
  CT2 : Inport
  F2 : Inport  Port=2
  E2 : Inport  Port=3
  MR2 : Inport  Port=4
  T2 : Inport  Port=5
  EB2 : Inport  Port=6
  CT3 : Inport  Port=7
  F3 : Inport  Port=8
  E3 : Inport  Port=9
  MR3 : Inport  Port=10
  T3 : Inport  Port=11
  EB3 : Inport  Port=12
  Tank2 : Subsystem
  Tank3 : Subsystem
  LL2 : Outport
  LL3 : Outport  Port=2
  wires:
  Tank2/1(LL2) -> LL2/1, Tank3/7(LL2)
  Tank3/1(LL3) -> LL3/1, Tank2/7(LL3)
  EB2/1 -> Tank2/6(EB2)
  MR3/1 -> Tank3/4(MR3)
  CT2/1 -> Tank2/1(CT2)
  F2/1 -> Tank2/2(F2)
  E3/1 -> Tank3/3(E3)
  E2/1 -> Tank2/3(E2)
  T2/1 -> Tank2/5(T2)
  CT3/1 -> Tank3/1(CT3)
  F3/1 -> Tank3/2(F3)
  EB3/1 -> Tank3/6(EB3)
  T3/1 -> Tank3/5(T3)
  MR2/1 -> Tank2/4(MR2)

== system c00006M_harness/M127 ==
  note: VALUES
      | ---------------------------------
      | ControlType = 1 | 2 | 3
      | FillTank = 0 | 1
      | EmptyTank = 0 | 1
      | ManualReference between 0 and 1
      | Tempreature between 0 and 100
      | EmergencyButton = 0 | 1
      | LiquidLevel between 0 and 1 (hmax)
  note: Inputs For Tank2
  note: NAMES
      | --------------------------------------------
      | CT1 = ControlType Tank 1
      | F1 = Fill Tank 1
      | E1 = Empty Tank 1
      | MR1 = Manual Reference Tank1
      | T1 = Temperature Tank 1
      | EB1 = Emergency Button Tank 1
      | LL1 = Liquid Level 1
  note: Inputs For Tank3
  note: Inputs For Tank1
  CT2 : Inport
  F2 : Inport  Port=2
  E2 : Inport  Port=3
  MR2 : Inport  Port=4
  T2 : Inport  Port=5
  EB2 : Inport  Port=6
  CT3 : Inport  Port=7
  F3 : Inport  Port=8
  E3 : Inport  Port=9
  MR3 : Inport  Port=10
  T3 : Inport  Port=11
  EB3 : Inport  Port=12
  Tank2 : Subsystem
  Tank3 : Subsystem
  LL2 : Outport
  LL3 : Outport  Port=2
  wires:
  Tank2/1(LL2) -> LL2/1, Tank3/7(LL2)
  Tank3/1(LL3) -> LL3/1, Tank2/7(LL3)
  EB2/1 -> Tank2/6(EB2)
  MR3/1 -> Tank3/4(MR3)
  CT2/1 -> Tank2/1(CT2)
  F2/1 -> Tank2/2(F2)
  E3/1 -> Tank3/3(E3)
  E2/1 -> Tank2/3(E2)
  T2/1 -> Tank2/5(T2)
  CT3/1 -> Tank3/1(CT3)
  F3/1 -> Tank3/2(F3)
  EB3/1 -> Tank3/6(EB3)
  T3/1 -> Tank3/5(T3)
  MR2/1 -> Tank2/4(MR2)

== system c00006M_harness/M128 ==
  note: VALUES
      | ---------------------------------
      | ControlType = 1 | 2 | 3
      | FillTank = 0 | 1
      | EmptyTank = 0 | 1
      | ManualReference between 0 and 1
      | Tempreature between 0 and 100
      | EmergencyButton = 0 | 1
      | LiquidLevel between 0 and 1 (hmax)
  note: Inputs For Tank2
  note: NAMES
      | --------------------------------------------
      | CT1 = ControlType Tank 1
      | F1 = Fill Tank 1
      | E1 = Empty Tank 1
      | MR1 = Manual Reference Tank1
      | T1 = Temperature Tank 1
      | EB1 = Emergency Button Tank 1
      | LL1 = Liquid Level 1
  note: Inputs For Tank3
  note: Inputs For Tank1
  CT2 : Inport
  F2 : Inport  Port=2
  E2 : Inport  Port=3
  MR2 : Inport  Port=4
  T2 : Inport  Port=5
  EB2 : Inport  Port=6
  CT3 : Inport  Port=7
  F3 : Inport  Port=8
  E3 : Inport  Port=9
  MR3 : Inport  Port=10
  T3 : Inport  Port=11
  EB3 : Inport  Port=12
  Tank2 : Subsystem
  Tank3 : Subsystem
  LL2 : Outport
  LL3 : Outport  Port=2
  wires:
  Tank2/1(LL2) -> LL2/1, Tank3/7(LL2)
  Tank3/1(LL3) -> LL3/1, Tank2/7(LL3)
  EB2/1 -> Tank2/6(EB2)
  MR3/1 -> Tank3/4(MR3)
  CT2/1 -> Tank2/1(CT2)
  F2/1 -> Tank2/2(F2)
  E3/1 -> Tank3/3(E3)
  E2/1 -> Tank2/3(E2)
  T2/1 -> Tank2/5(T2)
  CT3/1 -> Tank3/1(CT3)
  F3/1 -> Tank3/2(F3)
  EB3/1 -> Tank3/6(EB3)
  T3/1 -> Tank3/5(T3)
  MR2/1 -> Tank2/4(MR2)

== system c00006M_harness/M129 ==
  note: VALUES
      | ---------------------------------
      | ControlType = 1 | 2 | 3
      | FillTank = 0 | 1
      | EmptyTank = 0 | 1
      | ManualReference between 0 and 1
      | Tempreature between 0 and 100
      | EmergencyButton = 0 | 1
      | LiquidLevel between 0 and 1 (hmax)
  note: Inputs For Tank2
  note: NAMES
      | --------------------------------------------
      | CT1 = ControlType Tank 1
      | F1 = Fill Tank 1
      | E1 = Empty Tank 1
      | MR1 = Manual Reference Tank1
      | T1 = Temperature Tank 1
      | EB1 = Emergency Button Tank 1
      | LL1 = Liquid Level 1
  note: Inputs For Tank3
  note: Inputs For Tank1
  CT2 : Inport
  F2 : Inport  Port=2
  E2 : Inport  Port=3
  MR2 : Inport  Port=4
  T2 : Inport  Port=5
  EB2 : Inport  Port=6
  CT3 : Inport  Port=7
  F3 : Inport  Port=8
  E3 : Inport  Port=9
  MR3 : Inport  Port=10
  T3 : Inport  Port=11
  EB3 : Inport  Port=12
  Tank2 : Subsystem
  Tank3 : Subsystem
  LL2 : Outport
  LL3 : Outport  Port=2
  wires:
  Tank2/1(LL2) -> LL2/1, Tank3/7(LL2)
  Tank3/1(LL3) -> LL3/1, Tank2/7(LL3)
  EB2/1 -> Tank2/6(EB2)
  MR3/1 -> Tank3/4(MR3)
  CT2/1 -> Tank2/1(CT2)
  F2/1 -> Tank2/2(F2)
  E3/1 -> Tank3/3(E3)
  E2/1 -> Tank2/3(E2)
  T2/1 -> Tank2/5(T2)
  CT3/1 -> Tank3/1(CT3)
  F3/1 -> Tank3/2(F3)
  EB3/1 -> Tank3/6(EB3)
  T3/1 -> Tank3/5(T3)
  MR2/1 -> Tank2/4(MR2)

== system c00006M_harness/M130 ==
  note: VALUES
      | ---------------------------------
      | ControlType = 1 | 2 | 3
      | FillTank = 0 | 1
      | EmptyTank = 0 | 1
      | ManualReference between 0 and 1
      | Tempreature between 0 and 100
      | EmergencyButton = 0 | 1
      | LiquidLevel between 0 and 1 (hmax)
  note: Inputs For Tank2
  note: NAMES
      | --------------------------------------------
      | CT1 = ControlType Tank 1
      | F1 = Fill Tank 1
      | E1 = Empty Tank 1
      | MR1 = Manual Reference Tank1
      | T1 = Temperature Tank 1
      | EB1 = Emergency Button Tank 1
      | LL1 = Liquid Level 1
  note: Inputs For Tank3
  note: Inputs For Tank1
  CT2 : Inport
  F2 : Inport  Port=2
  E2 : Inport  Port=3
  MR2 : Inport  Port=4
  T2 : Inport  Port=5
  EB2 : Inport  Port=6
  CT3 : Inport  Port=7
  F3 : Inport  Port=8
  E3 : Inport  Port=9
  MR3 : Inport  Port=10
  T3 : Inport  Port=11
  EB3 : Inport  Port=12
  Tank2 : Subsystem
  Tank3 : Subsystem
  LL2 : Outport
  LL3 : Outport  Port=2
  wires:
  Tank2/1(LL2) -> LL2/1, Tank3/7(LL2)
  Tank3/1(LL3) -> LL3/1, Tank2/7(LL3)
  EB2/1 -> Tank2/6(EB2)
  MR3/1 -> Tank3/4(MR3)
  CT2/1 -> Tank2/1(CT2)
  F2/1 -> Tank2/2(F2)
  E3/1 -> Tank3/3(E3)
  E2/1 -> Tank2/3(E2)
  T2/1 -> Tank2/5(T2)
  CT3/1 -> Tank3/1(CT3)
  F3/1 -> Tank3/2(F3)
  EB3/1 -> Tank3/6(EB3)
  T3/1 -> Tank3/5(T3)
  MR2/1 -> Tank2/4(MR2)

== system c00006M_harness/M131 ==
  note: VALUES
      | ---------------------------------
      | ControlType = 1 | 2 | 3
      | FillTank = 0 | 1
      | EmptyTank = 0 | 1
      | ManualReference between 0 and 1
      | Tempreature between 0 and 100
      | EmergencyButton = 0 | 1
      | LiquidLevel between 0 and 1 (hmax)
  note: Inputs For Tank2
  note: NAMES
      | --------------------------------------------
      | CT1 = ControlType Tank 1
      | F1 = Fill Tank 1
      | E1 = Empty Tank 1
      | MR1 = Manual Reference Tank1
      | T1 = Temperature Tank 1
      | EB1 = Emergency Button Tank 1
      | LL1 = Liquid Level 1
  note: Inputs For Tank3
  note: Inputs For Tank1
  CT2 : Inport
  F2 : Inport  Port=2
  E2 : Inport  Port=3
  MR2 : Inport  Port=4
  T2 : Inport  Port=5
  EB2 : Inport  Port=6
  CT3 : Inport  Port=7
  F3 : Inport  Port=8
  E3 : Inport  Port=9
  MR3 : Inport  Port=10
  T3 : Inport  Port=11
  EB3 : Inport  Port=12
  Tank2 : Subsystem
  Tank3 : Subsystem
  LL2 : Outport
  LL3 : Outport  Port=2
  wires:
  Tank2/1(LL2) -> LL2/1, Tank3/7(LL2)
  Tank3/1(LL3) -> LL3/1, Tank2/7(LL3)
  EB2/1 -> Tank2/6(EB2)
  MR3/1 -> Tank3/4(MR3)
  CT2/1 -> Tank2/1(CT2)
  F2/1 -> Tank2/2(F2)
  E3/1 -> Tank3/3(E3)
  E2/1 -> Tank2/3(E2)
  T2/1 -> Tank2/5(T2)
  CT3/1 -> Tank3/1(CT3)
  F3/1 -> Tank3/2(F3)
  EB3/1 -> Tank3/6(EB3)
  T3/1 -> Tank3/5(T3)
  MR2/1 -> Tank2/4(MR2)

== system c00006M_harness/M132 ==
  note: VALUES
      | ---------------------------------
      | ControlType = 1 | 2 | 3
      | FillTank = 0 | 1
      | EmptyTank = 0 | 1
      | ManualReference between 0 and 1
      | Tempreature between 0 and 100
      | EmergencyButton = 0 | 1
      | LiquidLevel between 0 and 1 (hmax)
  note: Inputs For Tank2
  note: NAMES
      | --------------------------------------------
      | CT1 = ControlType Tank 1
      | F1 = Fill Tank 1
      | E1 = Empty Tank 1
      | MR1 = Manual Reference Tank1
      | T1 = Temperature Tank 1
      | EB1 = Emergency Button Tank 1
      | LL1 = Liquid Level 1
  note: Inputs For Tank3
  note: Inputs For Tank1
  CT2 : Inport
  F2 : Inport  Port=2
  E2 : Inport  Port=3
  MR2 : Inport  Port=4
  T2 : Inport  Port=5
  EB2 : Inport  Port=6
  CT3 : Inport  Port=7
  F3 : Inport  Port=8
  E3 : Inport  Port=9
  MR3 : Inport  Port=10
  T3 : Inport  Port=11
  EB3 : Inport  Port=12
  Tank2 : Subsystem
  Tank3 : Subsystem
  LL2 : Outport
  LL3 : Outport  Port=2
  wires:
  Tank2/1(LL2) -> LL2/1, Tank3/7(LL2)
  Tank3/1(LL3) -> LL3/1, Tank2/7(LL3)
  EB2/1 -> Tank2/6(EB2)
  MR3/1 -> Tank3/4(MR3)
  CT2/1 -> Tank2/1(CT2)
  F2/1 -> Tank2/2(F2)
  E3/1 -> Tank3/3(E3)
  E2/1 -> Tank2/3(E2)
  T2/1 -> Tank2/5(T2)
  CT3/1 -> Tank3/1(CT3)
  F3/1 -> Tank3/2(F3)
  EB3/1 -> Tank3/6(EB3)
  T3/1 -> Tank3/5(T3)
  MR2/1 -> Tank2/4(MR2)

== system c00006M_harness/M133 ==
  note: VALUES
      | ---------------------------------
      | ControlType = 1 | 2 | 3
      | FillTank = 0 | 1
      | EmptyTank = 0 | 1
      | ManualReference between 0 and 1
      | Tempreature between 0 and 100
      | EmergencyButton = 0 | 1
      | LiquidLevel between 0 and 1 (hmax)
  note: Inputs For Tank2
  note: NAMES
      | --------------------------------------------
      | CT1 = ControlType Tank 1
      | F1 = Fill Tank 1
      | E1 = Empty Tank 1
      | MR1 = Manual Reference Tank1
      | T1 = Temperature Tank 1
      | EB1 = Emergency Button Tank 1
      | LL1 = Liquid Level 1
  note: Inputs For Tank3
  note: Inputs For Tank1
  CT2 : Inport
  F2 : Inport  Port=2
  E2 : Inport  Port=3
  MR2 : Inport  Port=4
  T2 : Inport  Port=5
  EB2 : Inport  Port=6
  CT3 : Inport  Port=7
  F3 : Inport  Port=8
  E3 : Inport  Port=9
  MR3 : Inport  Port=10
  T3 : Inport  Port=11
  EB3 : Inport  Port=12
  Tank2 : Subsystem
  Tank3 : Subsystem
  LL2 : Outport
  LL3 : Outport  Port=2
  wires:
  Tank2/1(LL2) -> LL2/1, Tank3/7(LL2)
  Tank3/1(LL3) -> LL3/1, Tank2/7(LL3)
  EB2/1 -> Tank2/6(EB2)
  MR3/1 -> Tank3/4(MR3)
  CT2/1 -> Tank2/1(CT2)
  F2/1 -> Tank2/2(F2)
  E3/1 -> Tank3/3(E3)
  E2/1 -> Tank2/3(E2)
  T2/1 -> Tank2/5(T2)
  CT3/1 -> Tank3/1(CT3)
  F3/1 -> Tank3/2(F3)
  EB3/1 -> Tank3/6(EB3)
  T3/1 -> Tank3/5(T3)
  MR2/1 -> Tank2/4(MR2)

== system c00006M_harness/M134 ==
  note: VALUES
      | ---------------------------------
      | ControlType = 1 | 2 | 3
      | FillTank = 0 | 1
      | EmptyTank = 0 | 1
      | ManualReference between 0 and 1
      | Tempreature between 0 and 100
      | EmergencyButton = 0 | 1
      | LiquidLevel between 0 and 1 (hmax)
  note: Inputs For Tank2
  note: NAMES
      | --------------------------------------------
      | CT1 = ControlType Tank 1
      | F1 = Fill Tank 1
      | E1 = Empty Tank 1
      | MR1 = Manual Reference Tank1
      | T1 = Temperature Tank 1
      | EB1 = Emergency Button Tank 1
      | LL1 = Liquid Level 1
  note: Inputs For Tank3
  note: Inputs For Tank1
  CT2 : Inport
  F2 : Inport  Port=2
  E2 : Inport  Port=3
  MR2 : Inport  Port=4
  T2 : Inport  Port=5
  EB2 : Inport  Port=6
  CT3 : Inport  Port=7
  F3 : Inport  Port=8
  E3 : Inport  Port=9
  MR3 : Inport  Port=10
  T3 : Inport  Port=11
  EB3 : Inport  Port=12
  Tank2 : Subsystem
  Tank3 : Subsystem
  LL2 : Outport
  LL3 : Outport  Port=2
  wires:
  Tank2/1(LL2) -> LL2/1, Tank3/7(LL2)
  Tank3/1(LL3) -> LL3/1, Tank2/7(LL3)
  EB2/1 -> Tank2/6(EB2)
  MR3/1 -> Tank3/4(MR3)
  CT2/1 -> Tank2/1(CT2)
  F2/1 -> Tank2/2(F2)
  E3/1 -> Tank3/3(E3)
  E2/1 -> Tank2/3(E2)
  T2/1 -> Tank2/5(T2)
  CT3/1 -> Tank3/1(CT3)
  F3/1 -> Tank3/2(F3)
  EB3/1 -> Tank3/6(EB3)
  T3/1 -> Tank3/5(T3)
  MR2/1 -> Tank2/4(MR2)

== system c00006M_harness/M135 ==
  note: VALUES
      | ---------------------------------
      | ControlType = 1 | 2 | 3
      | FillTank = 0 | 1
      | EmptyTank = 0 | 1
      | ManualReference between 0 and 1
      | Tempreature between 0 and 100
      | EmergencyButton = 0 | 1
      | LiquidLevel between 0 and 1 (hmax)
  note: Inputs For Tank2
  note: NAMES
      | --------------------------------------------
      | CT1 = ControlType Tank 1
      | F1 = Fill Tank 1
      | E1 = Empty Tank 1
      | MR1 = Manual Reference Tank1
      | T1 = Temperature Tank 1
      | EB1 = Emergency Button Tank 1
      | LL1 = Liquid Level 1
  note: Inputs For Tank3
  note: Inputs For Tank1
  CT2 : Inport
  F2 : Inport  Port=2
  E2 : Inport  Port=3
  MR2 : Inport  Port=4
  T2 : Inport  Port=5
  EB2 : Inport  Port=6
  CT3 : Inport  Port=7
  F3 : Inport  Port=8
  E3 : Inport  Port=9
  MR3 : Inport  Port=10
  T3 : Inport  Port=11
  EB3 : Inport  Port=12
  Tank2 : Subsystem
  Tank3 : Subsystem
  LL2 : Outport
  LL3 : Outport  Port=2
  wires:
  Tank2/1(LL2) -> LL2/1, Tank3/7(LL2)
  Tank3/1(LL3) -> LL3/1, Tank2/7(LL3)
  EB2/1 -> Tank2/6(EB2)
  MR3/1 -> Tank3/4(MR3)
  CT2/1 -> Tank2/1(CT2)
  F2/1 -> Tank2/2(F2)
  E3/1 -> Tank3/3(E3)
  E2/1 -> Tank2/3(E2)
  T2/1 -> Tank2/5(T2)
  CT3/1 -> Tank3/1(CT3)
  F3/1 -> Tank3/2(F3)
  EB3/1 -> Tank3/6(EB3)
  T3/1 -> Tank3/5(T3)
  MR2/1 -> Tank2/4(MR2)

== system c00006M_harness/M136 ==
  note: VALUES
      | ---------------------------------
      | ControlType = 1 | 2 | 3
      | FillTank = 0 | 1
      | EmptyTank = 0 | 1
      | ManualReference between 0 and 1
      | Tempreature between 0 and 100
      | EmergencyButton = 0 | 1
      | LiquidLevel between 0 and 1 (hmax)
  note: Inputs For Tank2
  note: NAMES
      | --------------------------------------------
      | CT1 = ControlType Tank 1
      | F1 = Fill Tank 1
      | E1 = Empty Tank 1
      | MR1 = Manual Reference Tank1
      | T1 = Temperature Tank 1
      | EB1 = Emergency Button Tank 1
      | LL1 = Liquid Level 1
  note: Inputs For Tank3
  note: Inputs For Tank1
  CT2 : Inport
  F2 : Inport  Port=2
  E2 : Inport  Port=3
  MR2 : Inport  Port=4
  T2 : Inport  Port=5
  EB2 : Inport  Port=6
  CT3 : Inport  Port=7
  F3 : Inport  Port=8
  E3 : Inport  Port=9
  MR3 : Inport  Port=10
  T3 : Inport  Port=11
  EB3 : Inport  Port=12
  Tank2 : Subsystem
  Tank3 : Subsystem
  LL2 : Outport
  LL3 : Outport  Port=2
  wires:
  Tank2/1(LL2) -> LL2/1, Tank3/7(LL2)
  Tank3/1(LL3) -> LL3/1, Tank2/7(LL3)
  EB2/1 -> Tank2/6(EB2)
  MR3/1 -> Tank3/4(MR3)
  CT2/1 -> Tank2/1(CT2)
  F2/1 -> Tank2/2(F2)
  E3/1 -> Tank3/3(E3)
  E2/1 -> Tank2/3(E2)
  T2/1 -> Tank2/5(T2)
  CT3/1 -> Tank3/1(CT3)
  F3/1 -> Tank3/2(F3)
  EB3/1 -> Tank3/6(EB3)
  T3/1 -> Tank3/5(T3)
  MR2/1 -> Tank2/4(MR2)

== system c00006M_harness/M137 ==
  note: VALUES
      | ---------------------------------
      | ControlType = 1 | 2 | 3
      | FillTank = 0 | 1
      | EmptyTank = 0 | 1
      | ManualReference between 0 and 1
      | Tempreature between 0 and 100
      | EmergencyButton = 0 | 1
      | LiquidLevel between 0 and 1 (hmax)
  note: Inputs For Tank2
  note: NAMES
      | --------------------------------------------
      | CT1 = ControlType Tank 1
      | F1 = Fill Tank 1
      | E1 = Empty Tank 1
      | MR1 = Manual Reference Tank1
      | T1 = Temperature Tank 1
      | EB1 = Emergency Button Tank 1
      | LL1 = Liquid Level 1
  note: Inputs For Tank3
  note: Inputs For Tank1
  CT2 : Inport
  F2 : Inport  Port=2
  E2 : Inport  Port=3
  MR2 : Inport  Port=4
  T2 : Inport  Port=5
  EB2 : Inport  Port=6
  CT3 : Inport  Port=7
  F3 : Inport  Port=8
  E3 : Inport  Port=9
  MR3 : Inport  Port=10
  T3 : Inport  Port=11
  EB3 : Inport  Port=12
  Tank2 : Subsystem
  Tank3 : Subsystem
  LL2 : Outport
  LL3 : Outport  Port=2
  wires:
  Tank2/1(LL2) -> LL2/1, Tank3/7(LL2)
  Tank3/1(LL3) -> LL3/1, Tank2/7(LL3)
  EB2/1 -> Tank2/6(EB2)
  MR3/1 -> Tank3/4(MR3)
  CT2/1 -> Tank2/1(CT2)
  F2/1 -> Tank2/2(F2)
  E3/1 -> Tank3/3(E3)
  E2/1 -> Tank2/3(E2)
  T2/1 -> Tank2/5(T2)
  CT3/1 -> Tank3/1(CT3)
  F3/1 -> Tank3/2(F3)
  EB3/1 -> Tank3/6(EB3)
  T3/1 -> Tank3/5(T3)
  MR2/1 -> Tank2/4(MR2)

== system c00006M_harness/M138 ==
  note: VALUES
      | ---------------------------------
      | ControlType = 1 | 2 | 3
      | FillTank = 0 | 1
      | EmptyTank = 0 | 1
      | ManualReference between 0 and 1
      | Tempreature between 0 and 100
      | EmergencyButton = 0 | 1
      | LiquidLevel between 0 and 1 (hmax)
  note: Inputs For Tank2
  note: NAMES
      | --------------------------------------------
      | CT1 = ControlType Tank 1
      | F1 = Fill Tank 1
      | E1 = Empty Tank 1
      | MR1 = Manual Reference Tank1
      | T1 = Temperature Tank 1
      | EB1 = Emergency Button Tank 1
      | LL1 = Liquid Level 1
  note: Inputs For Tank3
  note: Inputs For Tank1
  CT2 : Inport
  F2 : Inport  Port=2
  E2 : Inport  Port=3
  MR2 : Inport  Port=4
  T2 : Inport  Port=5
  EB2 : Inport  Port=6
  CT3 : Inport  Port=7
  F3 : Inport  Port=8
  E3 : Inport  Port=9
  MR3 : Inport  Port=10
  T3 : Inport  Port=11
  EB3 : Inport  Port=12
  Tank2 : Subsystem
  Tank3 : Subsystem
  LL2 : Outport
  LL3 : Outport  Port=2
  wires:
  Tank2/1(LL2) -> LL2/1, Tank3/7(LL2)
  Tank3/1(LL3) -> LL3/1, Tank2/7(LL3)
  EB2/1 -> Tank2/6(EB2)
  MR3/1 -> Tank3/4(MR3)
  CT2/1 -> Tank2/1(CT2)
  F2/1 -> Tank2/2(F2)
  E3/1 -> Tank3/3(E3)
  E2/1 -> Tank2/3(E2)
  T2/1 -> Tank2/5(T2)
  CT3/1 -> Tank3/1(CT3)
  F3/1 -> Tank3/2(F3)
  EB3/1 -> Tank3/6(EB3)
  T3/1 -> Tank3/5(T3)
  MR2/1 -> Tank2/4(MR2)

== system c00006M_harness/M139 ==
  note: VALUES
      | ---------------------------------
      | ControlType = 1 | 2 | 3
      | FillTank = 0 | 1
      | EmptyTank = 0 | 1
      | ManualReference between 0 and 1
      | Tempreature between 0 and 100
      | EmergencyButton = 0 | 1
      | LiquidLevel between 0 and 1 (hmax)
  note: Inputs For Tank2
  note: NAMES
      | --------------------------------------------
      | CT1 = ControlType Tank 1
      | F1 = Fill Tank 1
      | E1 = Empty Tank 1
      | MR1 = Manual Reference Tank1
      | T1 = Temperature Tank 1
      | EB1 = Emergency Button Tank 1
      | LL1 = Liquid Level 1
  note: Inputs For Tank3
  note: Inputs For Tank1
  CT2 : Inport
  F2 : Inport  Port=2
  E2 : Inport  Port=3
  MR2 : Inport  Port=4
  T2 : Inport  Port=5
  EB2 : Inport  Port=6
  CT3 : Inport  Port=7
  F3 : Inport  Port=8
  E3 : Inport  Port=9
  MR3 : Inport  Port=10
  T3 : Inport  Port=11
  EB3 : Inport  Port=12
  Tank2 : Subsystem
  Tank3 : Subsystem
  LL2 : Outport
  LL3 : Outport  Port=2
  wires:
  Tank2/1(LL2) -> LL2/1, Tank3/7(LL2)
  Tank3/1(LL3) -> LL3/1, Tank2/7(LL3)
  EB2/1 -> Tank2/6(EB2)
  MR3/1 -> Tank3/4(MR3)
  CT2/1 -> Tank2/1(CT2)
  F2/1 -> Tank2/2(F2)
  E3/1 -> Tank3/3(E3)
  E2/1 -> Tank2/3(E2)
  T2/1 -> Tank2/5(T2)
  CT3/1 -> Tank3/1(CT3)
  F3/1 -> Tank3/2(F3)
  EB3/1 -> Tank3/6(EB3)
  T3/1 -> Tank3/5(T3)
  MR2/1 -> Tank2/4(MR2)

== system c00006M_harness/M140 ==
  note: VALUES
      | ---------------------------------
      | ControlType = 1 | 2 | 3
      | FillTank = 0 | 1
      | EmptyTank = 0 | 1
      | ManualReference between 0 and 1
      | Tempreature between 0 and 100
      | EmergencyButton = 0 | 1
      | LiquidLevel between 0 and 1 (hmax)
  note: Inputs For Tank2
  note: NAMES
      | --------------------------------------------
      | CT1 = ControlType Tank 1
      | F1 = Fill Tank 1
      | E1 = Empty Tank 1
      | MR1 = Manual Reference Tank1
      | T1 = Temperature Tank 1
      | EB1 = Emergency Button Tank 1
      | LL1 = Liquid Level 1
  note: Inputs For Tank3
  note: Inputs For Tank1
  CT2 : Inport
  F2 : Inport  Port=2
  E2 : Inport  Port=3
  MR2 : Inport  Port=4
  T2 : Inport  Port=5
  EB2 : Inport  Port=6
  CT3 : Inport  Port=7
  F3 : Inport  Port=8
  E3 : Inport  Port=9
  MR3 : Inport  Port=10
  T3 : Inport  Port=11
  EB3 : Inport  Port=12
  Tank2 : Subsystem
  Tank3 : Subsystem
  LL2 : Outport
  LL3 : Outport  Port=2
  wires:
  Tank2/1(LL2) -> LL2/1, Tank3/7(LL2)
  Tank3/1(LL3) -> LL3/1, Tank2/7(LL3)
  EB2/1 -> Tank2/6(EB2)
  MR3/1 -> Tank3/4(MR3)
  CT2/1 -> Tank2/1(CT2)
  F2/1 -> Tank2/2(F2)
  E3/1 -> Tank3/3(E3)
  E2/1 -> Tank2/3(E2)
  T2/1 -> Tank2/5(T2)
  CT3/1 -> Tank3/1(CT3)
  F3/1 -> Tank3/2(F3)
  EB3/1 -> Tank3/6(EB3)
  T3/1 -> Tank3/5(T3)
  MR2/1 -> Tank2/4(MR2)

== system c00006M_harness/M141 ==
  note: VALUES
      | ---------------------------------
      | ControlType = 1 | 2 | 3
      | FillTank = 0 | 1
      | EmptyTank = 0 | 1
      | ManualReference between 0 and 1
      | Tempreature between 0 and 100
      | EmergencyButton = 0 | 1
      | LiquidLevel between 0 and 1 (hmax)
  note: Inputs For Tank2
  note: NAMES
      | --------------------------------------------
      | CT1 = ControlType Tank 1
      | F1 = Fill Tank 1
      | E1 = Empty Tank 1
      | MR1 = Manual Reference Tank1
      | T1 = Temperature Tank 1
      | EB1 = Emergency Button Tank 1
      | LL1 = Liquid Level 1
  note: Inputs For Tank3
  note: Inputs For Tank1
  CT2 : Inport
  F2 : Inport  Port=2
  E2 : Inport  Port=3
  MR2 : Inport  Port=4
  T2 : Inport  Port=5
  EB2 : Inport  Port=6
  CT3 : Inport  Port=7
  F3 : Inport  Port=8
  E3 : Inport  Port=9
  MR3 : Inport  Port=10
  T3 : Inport  Port=11
  EB3 : Inport  Port=12
  Tank2 : Subsystem
  Tank3 : Subsystem
  LL2 : Outport
  LL3 : Outport  Port=2
  wires:
  Tank2/1(LL2) -> LL2/1, Tank3/7(LL2)
  Tank3/1(LL3) -> LL3/1, Tank2/7(LL3)
  EB2/1 -> Tank2/6(EB2)
  MR3/1 -> Tank3/4(MR3)
  CT2/1 -> Tank2/1(CT2)
  F2/1 -> Tank2/2(F2)
  E3/1 -> Tank3/3(E3)
  E2/1 -> Tank2/3(E2)
  T2/1 -> Tank2/5(T2)
  CT3/1 -> Tank3/1(CT3)
  F3/1 -> Tank3/2(F3)
  EB3/1 -> Tank3/6(EB3)
  T3/1 -> Tank3/5(T3)
  MR2/1 -> Tank2/4(MR2)

== system c00006M_harness/M142 ==
  note: VALUES
      | ---------------------------------
      | ControlType = 1 | 2 | 3
      | FillTank = 0 | 1
      | EmptyTank = 0 | 1
      | ManualReference between 0 and 1
      | Tempreature between 0 and 100
      | EmergencyButton = 0 | 1
      | LiquidLevel between 0 and 1 (hmax)
  note: Inputs For Tank2
  note: NAMES
      | --------------------------------------------
      | CT1 = ControlType Tank 1
      | F1 = Fill Tank 1
      | E1 = Empty Tank 1
      | MR1 = Manual Reference Tank1
      | T1 = Temperature Tank 1
      | EB1 = Emergency Button Tank 1
      | LL1 = Liquid Level 1
  note: Inputs For Tank3
  note: Inputs For Tank1
  CT2 : Inport
  F2 : Inport  Port=2
  E2 : Inport  Port=3
  MR2 : Inport  Port=4
  T2 : Inport  Port=5
  EB2 : Inport  Port=6
  CT3 : Inport  Port=7
  F3 : Inport  Port=8
  E3 : Inport  Port=9
  MR3 : Inport  Port=10
  T3 : Inport  Port=11
  EB3 : Inport  Port=12
  Tank2 : Subsystem
  Tank3 : Subsystem
  LL2 : Outport
  LL3 : Outport  Port=2
  wires:
  Tank2/1(LL2) -> LL2/1, Tank3/7(LL2)
  Tank3/1(LL3) -> LL3/1, Tank2/7(LL3)
  EB2/1 -> Tank2/6(EB2)
  MR3/1 -> Tank3/4(MR3)
  CT2/1 -> Tank2/1(CT2)
  F2/1 -> Tank2/2(F2)
  E3/1 -> Tank3/3(E3)
  E2/1 -> Tank2/3(E2)
  T2/1 -> Tank2/5(T2)
  CT3/1 -> Tank3/1(CT3)
  F3/1 -> Tank3/2(F3)
  EB3/1 -> Tank3/6(EB3)
  T3/1 -> Tank3/5(T3)
  MR2/1 -> Tank2/4(MR2)

== system c00006M_harness/M143 ==
  note: VALUES
      | ---------------------------------
      | ControlType = 1 | 2 | 3
      | FillTank = 0 | 1
      | EmptyTank = 0 | 1
      | ManualReference between 0 and 1
      | Tempreature between 0 and 100
      | EmergencyButton = 0 | 1
      | LiquidLevel between 0 and 1 (hmax)
  note: Inputs For Tank2
  note: NAMES
      | --------------------------------------------
      | CT1 = ControlType Tank 1
      | F1 = Fill Tank 1
      | E1 = Empty Tank 1
      | MR1 = Manual Reference Tank1
      | T1 = Temperature Tank 1
      | EB1 = Emergency Button Tank 1
      | LL1 = Liquid Level 1
  note: Inputs For Tank3
  note: Inputs For Tank1
  CT2 : Inport
  F2 : Inport  Port=2
  E2 : Inport  Port=3
  MR2 : Inport  Port=4
  T2 : Inport  Port=5
  EB2 : Inport  Port=6
  CT3 : Inport  Port=7
  F3 : Inport  Port=8
  E3 : Inport  Port=9
  MR3 : Inport  Port=10
  T3 : Inport  Port=11
  EB3 : Inport  Port=12
  Tank2 : Subsystem
  Tank3 : Subsystem
  LL2 : Outport
  LL3 : Outport  Port=2
  wires:
  Tank2/1(LL2) -> LL2/1, Tank3/7(LL2)
  Tank3/1(LL3) -> LL3/1, Tank2/7(LL3)
  EB2/1 -> Tank2/6(EB2)
  MR3/1 -> Tank3/4(MR3)
  CT2/1 -> Tank2/1(CT2)
  F2/1 -> Tank2/2(F2)
  E3/1 -> Tank3/3(E3)
  E2/1 -> Tank2/3(E2)
  T2/1 -> Tank2/5(T2)
  CT3/1 -> Tank3/1(CT3)
  F3/1 -> Tank3/2(F3)
  EB3/1 -> Tank3/6(EB3)
  T3/1 -> Tank3/5(T3)
  MR2/1 -> Tank2/4(MR2)
